simulink model "cruise_control_PID"  (R2023b)
settings: Solver=VariableStepAuto  StartTime=0.0  StopTime=10.0  RelTol=1e-3
undefined symbols (not defined in the file): K1, K2, Kd, Kf, m1, m2
libraries: slpidlib x1
settings Model: Creator=au756794  LastModifiedBy=au756794

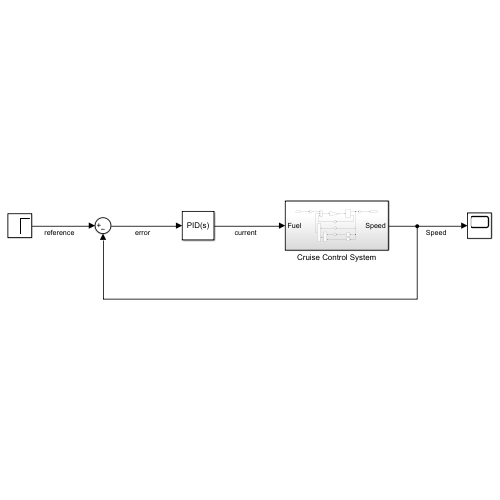
[thumbnail: Simulink's stored preview of the top-level diagram]
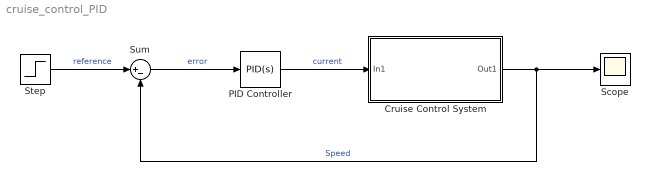
== system cruise_control_PID ==
  Cruise Control System : Subsystem
  PID Controller : slpidlib/PID Controller  Controller=PID  Form=Parallel  TimeDomain=Continuous-time  UseExternalTs=off  SampleTime=-1  IntegratorMethod=Forward Euler  FilterMethod=Forward Euler  ControllerParametersSource=internal  P=0.283977642795462  I=0.635522991115643  UseKiTs=off  D=0.0312131522452244  N=2489.98182340789  UseFilter=on  TunerSelectOption=Transfer Function Based (PID Tuner App)  InitialConditionSource=internal  InitialConditionForIntegrator=0  InitialConditionForFilter=0  DifferentiatorICPrevScaledInput=0  ExternalReset=none  TrackingMode=off  Kt=1  LimitOutput=off  SatLimitsSource=internal  UpperSaturationLimit=inf  LowerSaturationLimit=-inf  LinearizeAsGain=on  AntiWindupMode=none  Kb=1  LimitIntegrator=off  UpperIntegratorSaturationLimit=inf  LowerIntegratorSaturationLimit=-inf  POutMin=[]  POutMax=[]  IOutMin=[]  IOutMax=[]  DOutMin=[]  DOutMax=[]  NOutMin=[]  NOutMax=[]  SumOutMin=[]  SumOutMax=[]  SaturationOutMin=[]  SaturationOutMax=[]  PParamMin=[]  PParamMax=[]  IParamMin=[]  IParamMax=[]  DParamMin=[]  DParamMax=[]  NParamMin=[]  NParamMax=[]  KbParamMin=[]  KbParamMax=[]  KtParamMin=[]  KtParamMax=[]  KbOutMin=[]  KbOutMax=[]  KtOutMin=[]  KtOutMax=[]  IntegratorOutMin=[]  IntegratorOutMax=[]  FilterOutMin=[]  FilterOutMax=[]  SumI1OutMin=[]  SumI1OutMax=[]  SumI2OutMin=[]  SumI2OutMax=[]  SumI3OutMin=[]  SumI3OutMax=[]  SumI4OutMin=[]  SumI4OutMax=[]  SumDOutMin=[]  SumDOutMax=[]  DifferentiatorOutMin=[]  DifferentiatorOutMax=[]  FilterDiffOutCoefMin=[]  FilterDiffOutCoefMax=[]  ReciprocalOutMin=[]  ReciprocalOutMax=[]  SumDenOutMin=[]  SumDenOutMax=[]  SumNumOutMin=[]  SumNumOutMax=[]  DivideOutMin=[]  DivideOutMax=[]  UdiffTsProdOutMin=[]  UdiffTsProdOutMax=[]  NTsProdOutMin=[]  NTsProdOutMax=[]  UintegralTsProdOutMin=[]  UintegralTsProdOutMax=[]  UngainTsProdOutMin=[]  UngainTsProdOutMax=[]  ClampingZeroOutDataTypeStr=Inherit: Inherit via back propagation  ClampingZeroOutMin=[]  ClampingZeroOutMax=[]  FilterDenConstantOutDataTypeStr=Inherit: Inherit via back propagation  FilterDenConstantOutMin=[]  FilterDenConstantOutMax=[]  PCopyOutDataTypeStr=Inherit: Inherit via back propagation  PCopyOutMin=[]  PCopyOutMax=[]  NCopyOutDataTypeStr=Inherit: Inherit via back propagation  NCopyOutMin=[]  NCopyOutMax=[]  IntegratorContinuousStateAttributes=''  IntegratorStateMustResolveToSignalObject=off  IntegratorRTWStateStorageClass=Auto  FilterContinuousStateAttributes=''  FilterStateMustResolveToSignalObject=off  FilterRTWStateStorageClass=Auto  ParallelPVariant=InternalParameters  IdealPVariant=Disabled  IVariant=InternalParameters  DVariant=InternalParameters  IntegratorVariant=Continuous  SatVariant=Disabled  AWVariant=Passthrough  PCopyVariant=Disabled  TRVariant=Disabled  FdbkBlocksVariant=Forward  IdealPFdbkVariant=Disabled  SatFdbkVariant=Disabled  DerivativeFilterVariant=ContFilter  NVariant=InternalParameters  NCopyVariant=Disabled  FilterICVariant=InternalICsFilter  IntegratorICVariant=InternalICs  ExternalResetVariant=Disabled  TRSumVariant=Passthrough  SumFdbkVariant=Disabled  SumVariant=Sum_PID  TsampFilterVariant=InternalTs  TsampNgainVariant=Passthrough  TsampIntegralVariant=Disabled_SignalSpec  ExternalSaturationOutDataTypeStr=Inherit: Same as second input
  Scope : Scope
  Step : Step  After=15  SampleTime=0
  Sum : Sum  Inputs=|+-
  wires:
  PID Controller/1 -> Cruise Control System/1(In1)  "current"
  Sum/1 -> PID Controller/1  "error"
  Step/1 -> Sum/1  "reference"
  Cruise Control System/1(Out1) -> Scope/1, Sum/2  "Speed"

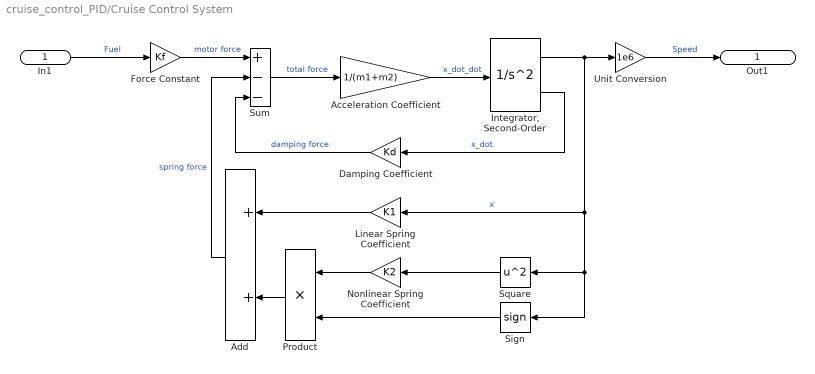
== system cruise_control_PID/Cruise Control System ==
  In1 : Inport
  Acceleration Coefficient : Gain  Gain=1/(m1+m2)
  Add : Sum
  Damping Coefficient : Gain  Gain=Kd
  Force Constant : Gain  Gain=Kf
  "Integrator, Second-Order" : SecondOrderIntegrator  ICX=0  LimitX=on  UpperLimitX=1e-3  LowerLimitX=0  IgnoreStateLimitsAndResetForLinearization=on
  Linear Spring Coefficient : Gain  Gain=K1
  Nonlinear Spring Coefficient : Gain  Gain=K2
  Product : Product
  Sign : Signum
  Square : Math  Operator=square
  Sum : Sum  Inputs=+--
  Unit Conversion : Gain  Gain=1e6
  Out1 : Outport
  wires:
  Unit Conversion/1 -> Out1/1  "Speed"
  In1/1 -> Force Constant/1  "Fuel"
  "Integrator, Second-Order"/2 -> Damping Coefficient/1  "x_dot"
  Sign/1 -> Product/2
  Sum/1 -> Acceleration Coefficient/1  "total force"
  Force Constant/1 -> Sum/1  "motor force"
  Acceleration Coefficient/1 -> "Integrator, Second-Order"/1  "x_dot_dot"
  Square/1 -> Nonlinear Spring Coefficient/1
  Damping Coefficient/1 -> Sum/3  "damping force"
  Linear Spring Coefficient/1 -> Add/1
  Nonlinear Spring Coefficient/1 -> Product/1
  Product/1 -> Add/2
  Add/1 -> Sum/2  "spring force"
  "Integrator, Second-Order"/1 -> Linear Spring Coefficient/1, Square/1, Sign/1, Unit Conversion/1  "x"
